simulink model "sampleModel154"  (R2021b)
settings: Solver=VariableStepAuto  StartTime=0.0  StopTime=10.0  RelTol=1e-3
undefined symbols (not defined in the file or in its folder): DiscIntNeverNeededParam, Newton, Raphson
libraries: simulink x4
settings Model: Creator=user  LastModifiedBy=user

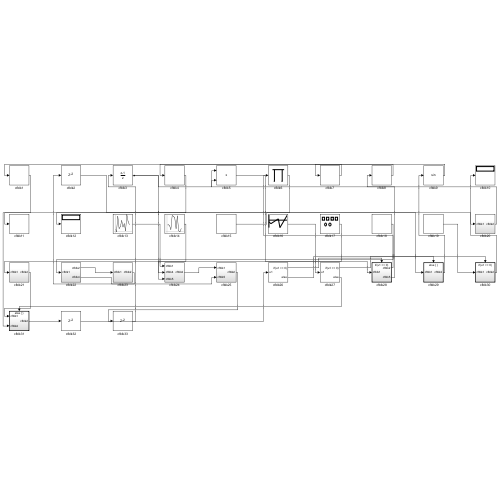
[thumbnail: Simulink's stored preview of the top-level diagram]
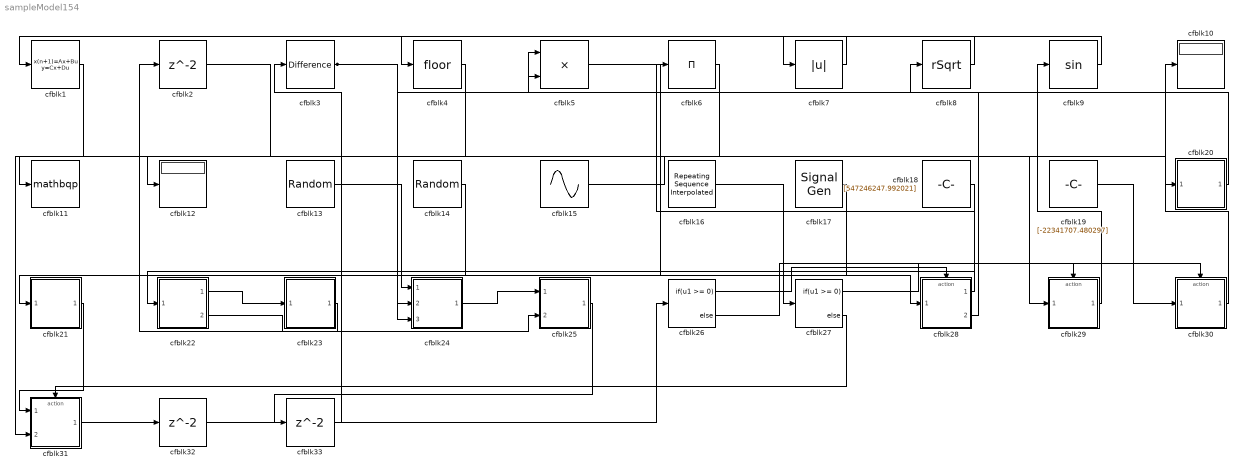
== system sampleModel154 ==
  cfblk1 : DiscreteStateSpace
  cfblk10 : Display
  cfblk11 : ToWorkspace  VariableName=mathbqp  SaveFormat=Timeseries  SampleTime=-1
  cfblk12 : Display
  cfblk13 : UniformRandomNumber  Minimum=[-421983085.608282]  Maximum=[3433340818.246167]  Seed=[66348310.000000]  SampleTime=0.1
  cfblk14 : RandomNumber  Mean=[-95778.519476]  Variance=[30138.949013]  Seed=[321896255.000000]  SampleTime=0.1
  cfblk15 : Sin  Amplitude=[638491597.447278]  Bias=[92663918.760373]  SampleTime=0
  cfblk16 : simulink/Sources/Repeating Sequence Interpolated  OutValues=[-205358164.498162, -482518571.738718, 186016604.222848, -986004521.728167, 721933685.230513]  TimeValues=[0 0.1 0.5 0.6 1].'  LookUpMeth=Use Input Below  tsamp=0.01  OutMin=[]  OutMax=[]  OutDataTypeStr=double  OutputDataTypeScalingMode=double  OutDataType=fixdt(0,8)  OutScaling=2^-10
  cfblk17 : SignalGenerator  Amplitude=[-48112224.356476]  Units=rad/sec
  cfblk18 : Constant  Value=[547246247.992021]  SampleTime=1
  cfblk19 : Constant  Value=[-22341707.480297]  SampleTime=1
  cfblk2 : Delay  SampleTime=1
  cfblk20 : Subsystem
  cfblk21 : Subsystem
  cfblk22 : Subsystem
  cfblk23 : Subsystem
  cfblk24 : Subsystem
  cfblk25 : Subsystem
  cfblk26 : If  IfExpression=u1 >= 0  SampleTime=1
  cfblk27 : If  IfExpression=u1 >= 0  SampleTime=1
  cfblk28 : Subsystem  TreatAsAtomicUnit=on
  cfblk29 : Subsystem  TreatAsAtomicUnit=on
  cfblk3 : simulink/Discrete/Difference  ICPrevInput=0.0  OutMin=[]  OutMax=[]  OutDataTypeStr=Inherit: Inherit via back propagation  OutDataType=fixdt(1, 16)  OutScaling=2^-10  DoSatur=off
  cfblk30 : Subsystem  TreatAsAtomicUnit=on
  cfblk31 : Subsystem  TreatAsAtomicUnit=on
  cfblk32 : Delay  SampleTime=1
  cfblk33 : Delay  SampleTime=1
  cfblk4 : Rounding
  cfblk5 : Product
  cfblk6 : Product  Inputs=*
  cfblk7 : Abs
  cfblk8 : Sqrt  Operator=rSqrt  AlgorithmType=Newton-Raphson  SaturateOnIntegerOverflow=on
  cfblk9 : Trigonometry
  wires:
  cfblk18/1 -> cfblk22/1(cfblk1)
  cfblk29/1(cfblk2) -> cfblk9/1
  cfblk24/1(cfblk2) -> cfblk25/1(cfblk1)
  cfblk15/1 -> cfblk29/1(cfblk1)
  cfblk23/1(cfblk2) -> cfblk2/1
  cfblk14/1 -> cfblk21/1(cfblk1)
  cfblk21/1(cfblk2) -> cfblk31/1(cfblk1)
  cfblk30/1(cfblk2) -> cfblk10/1
  cfblk13/1 -> cfblk24/1(cfblk1)
  cfblk8/1 -> cfblk4/1
  cfblk5/1 -> cfblk28/1(cfblk1)
  cfblk28/1(cfblk2) -> cfblk6/1
  cfblk7/1 -> cfblk1/1
  cfblk3/1 -> cfblk24/2(cfblk4), cfblk5/2
  cfblk6/1 -> cfblk31/2(cfblk4)
  cfblk16/1 -> cfblk27/1
  cfblk4/1 -> cfblk12/1
  cfblk28/2(cfblk5) -> cfblk8/1
  cfblk20/1(cfblk2) -> cfblk5/1
  cfblk9/1 -> cfblk7/1
  cfblk19/1 -> cfblk30/1(cfblk1)
  cfblk1/1 -> cfblk11/1
  cfblk22/1(cfblk2) -> cfblk23/1(cfblk1)
  cfblk22/2(cfblk4) -> cfblk25/2(cfblk5)
  cfblk17/1 -> cfblk24/3(cfblk5)
  cfblk2/1 -> cfblk20/1(cfblk1)
  cfblk26/1 -> cfblk28/Action
  cfblk26/2 -> cfblk29/Action
  cfblk27/1 -> cfblk30/Action
  cfblk27/2 -> cfblk31/Action
  cfblk31/1(cfblk2) -> cfblk32/1
  cfblk32/1 -> cfblk26/1
  cfblk25/1(cfblk2) -> cfblk33/1
  cfblk33/1 -> cfblk3/1

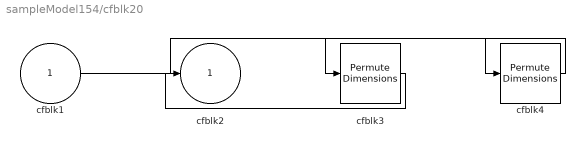
== system sampleModel154/cfblk20 ==
  cfblk1 : Inport
  cfblk3 : PermuteDimensions
  cfblk4 : PermuteDimensions
  cfblk2 : Outport
  wires:
  cfblk1/1 -> cfblk4/1
  cfblk3/1 -> cfblk2/1
  cfblk4/1 -> cfblk3/1

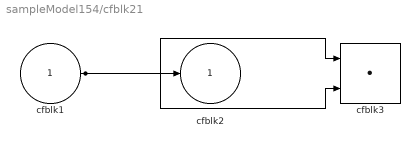
== system sampleModel154/cfblk21 ==
  cfblk1 : Inport
  cfblk3 : DotProduct  InputSameDT=on  OutDataTypeStr=Inherit: Inherit via internal rule
  cfblk2 : Outport
  wires:
  cfblk1/1 -> cfblk2/1, cfblk3/1, cfblk3/2

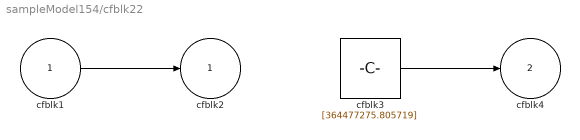
== system sampleModel154/cfblk22 ==
  cfblk1 : Inport
  cfblk3 : Constant  Value=[364477275.805719]  SampleTime=1
  cfblk2 : Outport
  cfblk4 : Outport  Port=2
  wires:
  cfblk1/1 -> cfblk2/1
  cfblk3/1 -> cfblk4/1

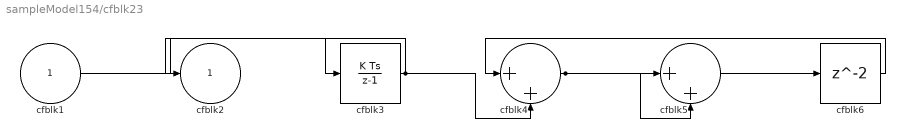
== system sampleModel154/cfblk23 ==
  cfblk1 : Inport
  cfblk3 : DiscreteIntegrator  ICPrevOutput=DiscIntNeverNeededParam  ICPrevScaledInput=DiscIntNeverNeededParam
  cfblk4 : Sum  Inputs=|++
  cfblk5 : Sum  Inputs=|++
  cfblk6 : Delay  SampleTime=1
  cfblk2 : Outport
  wires:
  cfblk3/1 -> cfblk4/2, cfblk2/1
  cfblk1/1 -> cfblk3/1
  cfblk4/1 -> cfblk5/1, cfblk5/2
  cfblk5/1 -> cfblk6/1
  cfblk6/1 -> cfblk4/1

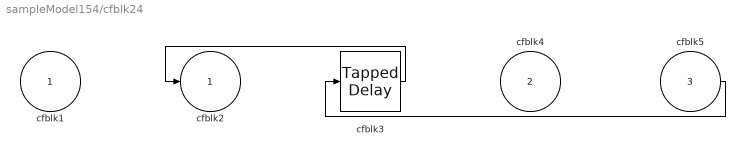
== system sampleModel154/cfblk24 ==
  cfblk1 : Inport
  cfblk4 : Inport  Port=2
  cfblk5 : Inport  Port=3
  cfblk3 : simulink/Discrete/Tapped Delay  vinit=0.0  samptime=-1  NumDelays=1  DelayOrder=Oldest  includeCurrent=off
  cfblk2 : Outport
  wires:
  cfblk3/1 -> cfblk2/1
  cfblk5/1 -> cfblk3/1

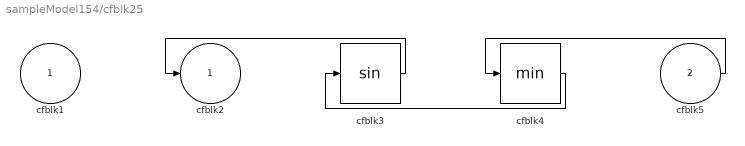
== system sampleModel154/cfblk25 ==
  cfblk1 : Inport
  cfblk5 : Inport  Port=2
  cfblk3 : Trigonometry
  cfblk4 : MinMax
  cfblk2 : Outport
  wires:
  cfblk3/1 -> cfblk2/1
  cfblk4/1 -> cfblk3/1
  cfblk5/1 -> cfblk4/1

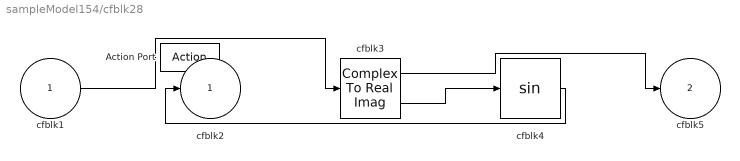
== system sampleModel154/cfblk28 ==
  cfblk1 : Inport
  Action Port : ActionPort  ActionPortLabel=if(u1 >= 0)
  cfblk3 : ComplexToRealImag
  cfblk4 : Trigonometry
  cfblk2 : Outport
  cfblk5 : Outport  Port=2
  wires:
  cfblk4/1 -> cfblk2/1
  cfblk1/1 -> cfblk3/1
  cfblk3/1 -> cfblk5/1
  cfblk3/2 -> cfblk4/1

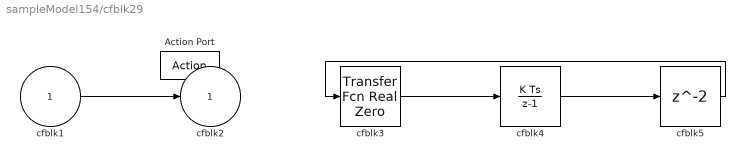
== system sampleModel154/cfblk29 ==
  cfblk1 : Inport
  Action Port : ActionPort  ActionPortLabel=else
  cfblk3 : simulink/Discrete/Transfer Fcn Real Zero  ZeroZ=0.75  ICPrevInput=0.0  DoSatur=off
      settings: SourceProductBaseCode=SL
  cfblk4 : DiscreteIntegrator  SampleTime=-1  ICPrevOutput=DiscIntNeverNeededParam  ICPrevScaledInput=DiscIntNeverNeededParam
  cfblk5 : Delay
  cfblk2 : Outport
  wires:
  cfblk3/1 -> cfblk4/1
  cfblk1/1 -> cfblk2/1
  cfblk4/1 -> cfblk5/1
  cfblk5/1 -> cfblk3/1

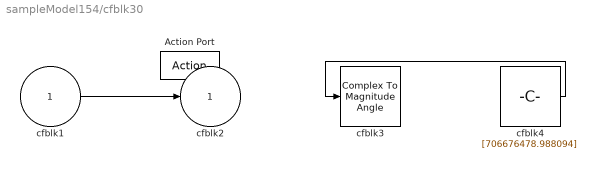
== system sampleModel154/cfblk30 ==
  cfblk1 : Inport
  Action Port : ActionPort  ActionPortLabel=if(u1 >= 0)
  cfblk3 : ComplexToMagnitudeAngle
  cfblk4 : Constant  Value=[706676478.988094]  SampleTime=1
  cfblk2 : Outport
  wires:
  cfblk1/1 -> cfblk2/1
  cfblk4/1 -> cfblk3/1

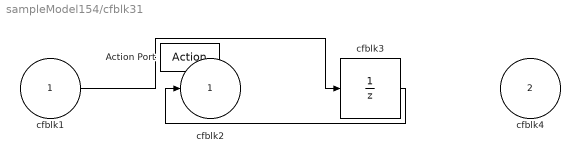
== system sampleModel154/cfblk31 ==
  cfblk1 : Inport
  cfblk4 : Inport  Port=2
  Action Port : ActionPort  ActionPortLabel=else
  cfblk3 : UnitDelay  SampleTime=-1  HasFrameUpgradeWarning=on
  cfblk2 : Outport
  wires:
  cfblk3/1 -> cfblk2/1
  cfblk1/1 -> cfblk3/1
